simulink model "test_plant"  (R2025a)
settings: Solver=VariableStepAuto  StartTime=0  StopTime=40  RelTol=1e-3
settings Model: Creator=techn  LastModifiedBy=techn

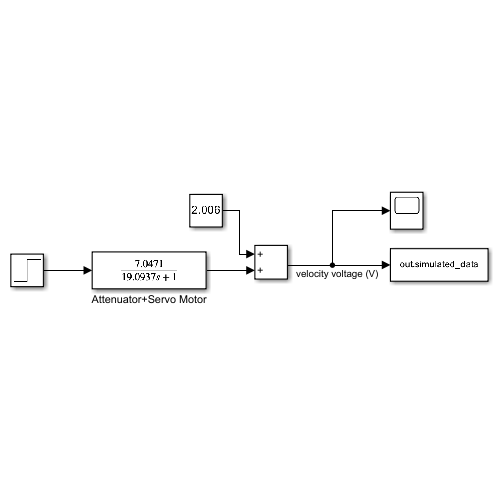
[thumbnail: Simulink's stored preview of the top-level diagram]
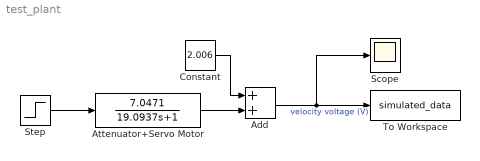
== system test_plant ==
  Add : Sum
  Attenuator+Servo Motor : TransferFcn  Numerator=7.0471  Denominator=[19.0937,1]
  Constant : Constant  Value=2.006
  Scope : Scope
      settings: ActiveDisplayYMinimum=-2.8444323936434337  ActiveDisplayYMaximum=17.746677545207294
  Step : Step  Time=25.7  After=0.5  SampleTime=0
  To Workspace : ToWorkspace  VariableName=simulated_data  SaveFormat=Timeseries  SampleTime=-1
  wires:
  Step/1 -> Attenuator+Servo Motor/1
  Add/1 -> To Workspace/1, Scope/1  "velocity voltage (V)"
  Attenuator+Servo Motor/1 -> Add/2
  Constant/1 -> Add/1
